simulink model "JSTraj"  (R2024b)
settings: Solver=ode8  StartTime=0.0  StopTime=Inf  FixedStep=0.001  RelTol=1e-3
model workspace (MAT data in the model file):
  q_init_l = Simulink.Parameter
  q_init_l.Value = [0.165747; 0.819274; 1.26369; 0.604148; 1.0515; -0.139217]
  q_init_l.Complexity = 'real'
  q_init_l.Dimensions = [6 1]
  q_init_l.DataType = 'double'
  q_init_r = Simulink.Parameter
  q_init_r.Value = [-0.165747; -0.819274; -1.26369; -0.604148; -1.0515; 0.139217]
  q_init_r.Complexity = 'real'
  q_init_r.Dimensions = [6 1]
  q_init_r.DataType = 'double'
  robot : robotics.RigidBodyTree (value not decoded)
libraries: robotcorelib x1
settings Model: Creator=sung  LastModifiedBy=sung
settings HardwareCC: ProdBitPerLong=64  ProdHWDeviceType=Intel->x86-64 (Linux 64)
settings RTWCC: GenCodeOnly=on  Toolchain=CMake

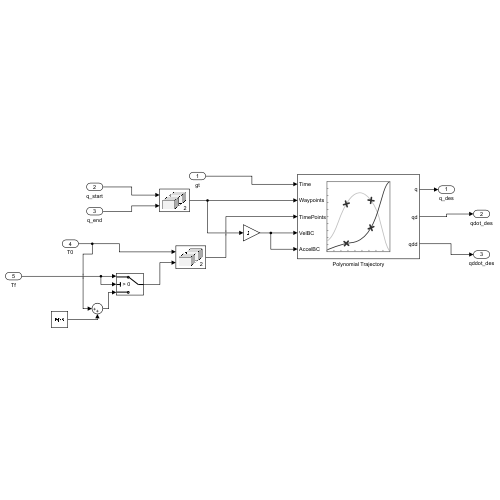
[thumbnail: Simulink's stored preview of the top-level diagram]
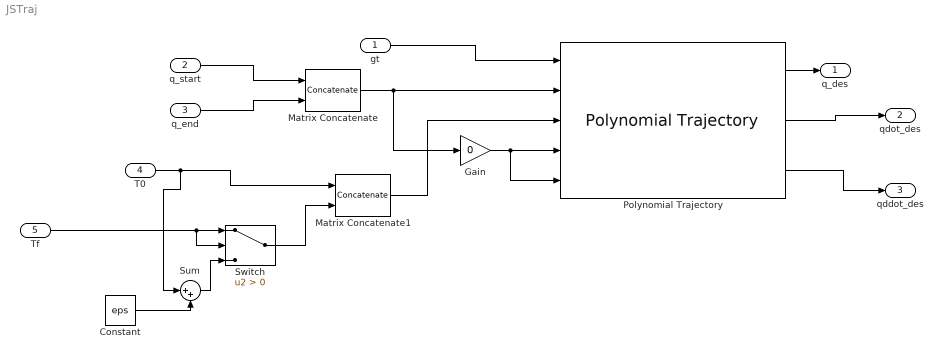
== system JSTraj ==
  gt : Inport
  q_start : Inport  Port=2  PortDimensions=6
  q_end : Inport  Port=3  PortDimensions=6
  T0 : Inport  Port=4
  Tf : Inport  Port=5  OutMin=[0.001]  OutMax=[1000]  OutDataTypeStr=double
  Constant : Constant  Value=eps
  Gain : Gain  Gain=0
  Matrix Concatenate : Concatenate  Mode=Multidimensional array  ConcatenateDimension=2
  Matrix Concatenate1 : Concatenate  Mode=Multidimensional array  ConcatenateDimension=2
  Polynomial Trajectory : robotcorelib/Polynomial Trajectory  WaypointSource=External  Waypoints=[ 0, 2, 1, 5, 0; -1, 3, 1, 4, 4 ]  TimePoints=[ 0, 1, 2, 3, 4 ]  TimeInterval=[ 1, 4 ]  Method=Quintic Polynomial  ParameterSource=External  VelocityBoundaryCondition=zeros( 2, 5 )  AccelerationBoundaryCondition=zeros( 2, 5 )  SimulateUsing=Code generation
  Sum : Sum  Inputs=|++
  Switch : Switch  Criteria=u2 > Threshold  SaturateOnIntegerOverflow=off  InputSameDT=off
  q_des : Outport
  qdot_des : Outport  Port=2
  qddot_des : Outport  Port=3
  wires:
  gt/1 -> Polynomial Trajectory/1
  Polynomial Trajectory/1 -> q_des/1
  Polynomial Trajectory/2 -> qdot_des/1
  Polynomial Trajectory/3 -> qddot_des/1
  q_start/1 -> Matrix Concatenate/1
  q_end/1 -> Matrix Concatenate/2
  Matrix Concatenate/1 -> Gain/1, Polynomial Trajectory/2
  Gain/1 -> Polynomial Trajectory/5, Polynomial Trajectory/4
  T0/1 -> Sum/1, Matrix Concatenate1/1
  Tf/1 -> Switch/2, Switch/1
  Matrix Concatenate1/1 -> Polynomial Trajectory/3
  Switch/1 -> Matrix Concatenate1/2
  Sum/1 -> Switch/3
  Constant/1 -> Sum/2
